simulink model "robust_defence_zda"  (R2022a)
settings: Solver=VariableStepAuto  StartTime=0.0  StopTime=6  RelTol=1e-3
values from neighbouring files (symbols this model uses):
  A = [zeros(3, 3) eye(3) ... (first row only)    [robust_defence_zda.m]
  A_obs1 = [-kappa1*c2   1 0 ... (first row only)    [robust_defence_zda.m]
  A_obs2 = [-kappa2*c2   1 0 ... (first row only)    [robust_defence_zda.m]
  A_obs3 = [-kappa3*c2   1 0 ... (first row only)    [robust_defence_zda.m]
  B = [zeros(3, 3); inv(M)]    [robust_defence_zda.m]
  b = Cp*(A^(r-1))*Bp    [robust_defence_zda.m]
  b0 = 62.5    [robust_defence_zda.m]
  B_obs = [0; b0; 0]    [robust_defence_zda.m]
  Cp = [0 0 1 0 0 0]    [robust_defence_zda.m]
  H0 = Cp*(A^r)*T0_inv    [robust_defence_zda.m]
  K = Cp*(A^r)*T1_inv    [robust_defence_zda.m]
  K0 = [-9 -6]    [robust_defence_zda.m]
  Ka = (-1)*acker(F0, G0a, [1/tau1 1/tau1 1/tau1 1/tau1])    [robust_defence_zda.m]
  kcr1 = [kappa1*c2; kappa1^2*c1; kappa1^3*c0]    [robust_defence_zda.m]
  kcr2 = [kappa2*c2; kappa2^2*c1; kappa2^3*c0]    [robust_defence_zda.m]
  kcr3 = [kappa3*c2; kappa3^2*c1; kappa3^3*c0]    [robust_defence_zda.m]
  L = 0.1    [robust_defence_zda.m]
  T0 = [1 0 0 0 0 0 ... (first row only)    [robust_defence_zda.m]
  T1 = [Cp; Cp*A]    [robust_defence_zda.m]
  x0 = [0; 0; 0; 0; omega20; 0]    [robust_defence_zda.m]
  xi_ext0 = [0; 0.085; 0.01]    [robust_defence_zda.m]
settings Model: Creator=edebi  LastModifiedBy=edebi

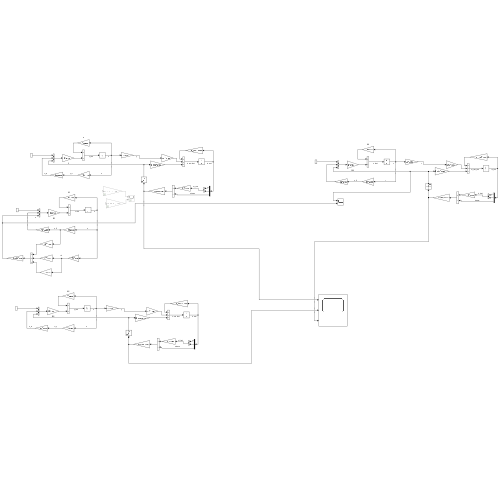
[thumbnail: Simulink's stored preview of the top-level diagram]
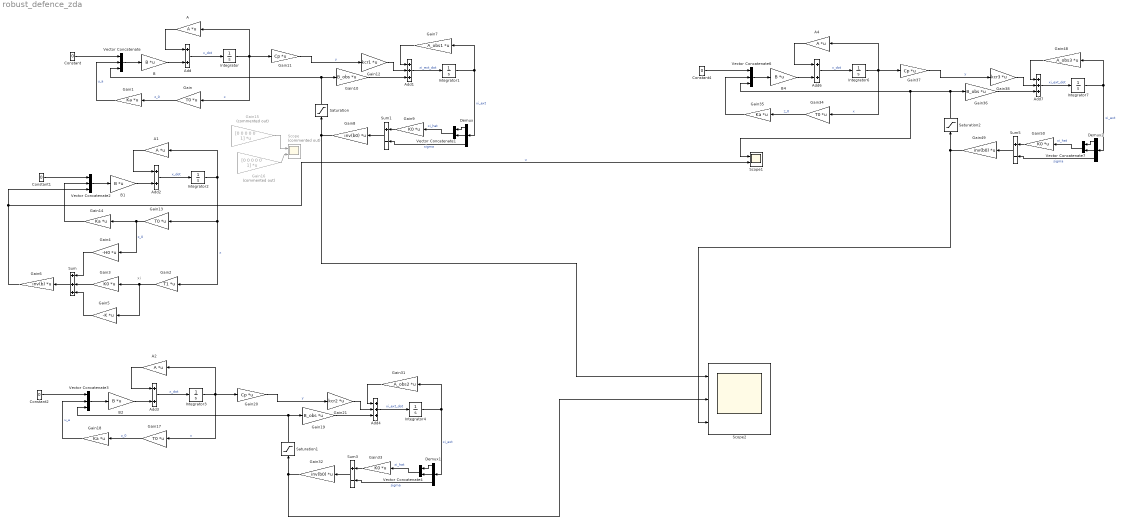
== system robust_defence_zda ==
  note: xi
  A{,1..2,4} (4 alike) : Gain  Gain=A  Multiplication=Matrix(K*u) (u vector)
  Add{,2..3,6} (4 alike) : Sum
  Add1 : Sum  Inputs=+++
  Add4 : Sum  Inputs=+++
  Add7 : Sum  Inputs=+++
  B{,1..2,4} (4 alike) : Gain  Gain=B  Multiplication=Matrix(K*u) (u vector)
  Constant{,1..2,4} (4 alike) : Constant  Value=0
  Demux : Demux  Outputs=3
  Demux1 : Demux  Outputs=3
  Demux2 : Demux  Outputs=3
  Gain{,13,17,34} (4 alike) : Gain  Gain=T0  Multiplication=Matrix(K*u) (u vector)
  Gain{1,14,18,35} (4 alike) : Gain  Gain=Ka  Multiplication=Matrix(K*u) (u vector)
  Gain10 : Gain  Gain=B_obs  Multiplication=Matrix(K*u) (u vector)
  Gain11 : Gain  Gain=Cp  Multiplication=Matrix(K*u) (u vector)
  Gain12 : Gain  Gain=kcr1  Multiplication=Matrix(K*u) (u vector)
  Gain15 : Gain  Commented=on  Gain=[0 0 0 0 0 1]  Multiplication=Matrix(K*u) (u vector)
  Gain16 : Gain  Commented=on  Gain=[0 0 0 0 0 1]  Multiplication=Matrix(K*u) (u vector)
  Gain19 : Gain  Gain=B_obs  Multiplication=Matrix(K*u) (u vector)
  Gain2 : Gain  Gain=T1  Multiplication=Matrix(K*u) (u vector)
  Gain20 : Gain  Gain=Cp  Multiplication=Matrix(K*u) (u vector)
  Gain21 : Gain  Gain=kcr2  Multiplication=Matrix(K*u) (u vector)
  Gain{3,9,33,50} (4 alike) : Gain  Gain=K0  Multiplication=Matrix(K*u) (u vector)
  Gain31 : Gain  Gain=A_obs2  Multiplication=Matrix(K*u) (u vector)
  Gain32 : Gain  Gain=inv(b0)  Multiplication=Matrix(K*u) (u vector)
  Gain36 : Gain  Gain=B_obs  Multiplication=Matrix(K*u) (u vector)
  Gain37 : Gain  Gain=Cp  Multiplication=Matrix(K*u) (u vector)
  Gain38 : Gain  Gain=kcr3  Multiplication=Matrix(K*u) (u vector)
  Gain4 : Gain  Gain=-H0  Multiplication=Matrix(K*u) (u vector)
  Gain48 : Gain  Gain=A_obs3  Multiplication=Matrix(K*u) (u vector)
  Gain49 : Gain  Gain=inv(b0)  Multiplication=Matrix(K*u) (u vector)
  Gain5 : Gain  Gain=-K  Multiplication=Matrix(K*u) (u vector)
  Gain6 : Gain  Gain=inv(b)  Multiplication=Matrix(K*u) (u vector)
  Gain7 : Gain  Gain=A_obs1  Multiplication=Matrix(K*u) (u vector)
  Gain8 : Gain  Gain=inv(b0)  Multiplication=Matrix(K*u) (u vector)
  Integrator{,2..3,6} (4 alike) : Integrator  InitialCondition=x0  ContinuousStateAttributes=['delta1' 'delta2' 'delta3' 'omega1' 'omega2' 'omega3']
  Integrator1 : Integrator  InitialCondition=xi_ext0
  Integrator4 : Integrator  InitialCondition=xi_ext0
  Integrator7 : Integrator  InitialCondition=xi_ext0
  Saturation : Saturate  UpperLimit=+L  LowerLimit=-L
  Saturation1 : Saturate  UpperLimit=+L  LowerLimit=-L
  Saturation2 : Saturate  UpperLimit=+L  LowerLimit=-L
  Scope : Scope  Commented=on  NumInputPorts=2
  Scope1 : Scope  NumInputPorts=2
  Scope2 : Scope  NumInputPorts=3
  Sum : Sum  Inputs=+++
  Sum1 : Sum  Inputs=+-
  Sum3 : Sum  Inputs=+-
  Sum5 : Sum  Inputs=+-
  Vector Concatenate{,2..3,6} (4 alike) : Concatenate  NumInputs=3
  Vector Concatenate1 : Concatenate
  Vector Concatenate4 : Concatenate
  Vector Concatenate7 : Concatenate
  wires:
  Constant/1 -> Vector Concatenate/1
  Sum/1 -> Gain6/1
  Gain5/1 -> Sum/3
  B/1 -> Add/2
  Gain1/1 -> Vector Concatenate/2  "u_a"
  Gain2/1 -> Gain5/1, Gain3/1
  Add/1 -> Integrator/1  "x_dot"
  Gain/1 -> Gain1/1  "z_0"
  Vector Concatenate/1 -> B/1
  Gain3/1 -> Sum/2
  Integrator/1 -> Gain/1, A/1, Gain11/1  "x"
  Gain4/1 -> Sum/1
  A/1 -> Add/1
  Add1/1 -> Integrator1/1  "xi_ext_dot"
  Gain7/1 -> Add1/1
  Demux/3 -> Sum1/2  "sigma"
  Gain9/1 -> Sum1/1
  Sum1/1 -> Gain8/1
  Gain11/1 -> Gain12/1  "y"
  Gain12/1 -> Add1/2
  Integrator1/1 -> Demux/1, Gain7/1  "xi_ext"
  Demux/2 -> Vector Concatenate1/2
  Demux/1 -> Vector Concatenate1/1
  Vector Concatenate1/1 -> Gain9/1  "xi_hat"
  Gain10/1 -> Add1/3
  Gain8/1 -> Saturation/1, Scope2/1
  Saturation/1 -> Gain10/1, Vector Concatenate/3
  Integrator2/1 -> Gain2/1, Gain13/1, A1/1  "x"
  Gain6/1 -> Scope1/2, Vector Concatenate2/3  "u"
  Gain14/1 -> Vector Concatenate2/2
  Gain13/1 -> Gain4/1, Gain14/1  "z_0"
  A1/1 -> Add2/1
  Vector Concatenate2/1 -> B1/1
  Add2/1 -> Integrator2/1  "x_dot"
  B1/1 -> Add2/2
  Constant1/1 -> Vector Concatenate2/1
  Gain15/1 -> Scope/1
  Gain16/1 -> Scope/2
  Gain20/1 -> Gain21/1  "y"
  Integrator4/1 -> Demux1/1, Gain31/1  "xi_ext"
  Add4/1 -> Integrator4/1  "xi_ext_dot"
  Saturation1/1 -> Gain19/1, Vector Concatenate3/3
  Gain19/1 -> Add4/3
  Demux1/2 -> Vector Concatenate4/2
  Demux1/1 -> Vector Concatenate4/1
  Integrator3/1 -> Gain17/1, A2/1, Gain20/1  "x"
  Gain33/1 -> Sum3/1
  Vector Concatenate3/1 -> B2/1
  Gain31/1 -> Add4/1
  Gain17/1 -> Gain18/1  "z_0"
  Gain18/1 -> Vector Concatenate3/2  "u_a"
  A2/1 -> Add3/1
  Gain21/1 -> Add4/2
  Add3/1 -> Integrator3/1  "x_dot"
  Gain32/1 -> Scope2/2, Saturation1/1
  Sum3/1 -> Gain32/1
  Demux1/3 -> Sum3/2  "sigma"
  Vector Concatenate4/1 -> Gain33/1  "xi_hat"
  B2/1 -> Add3/2
  Constant2/1 -> Vector Concatenate3/1
  Gain37/1 -> Gain38/1  "y"
  Integrator7/1 -> Demux2/1, Gain48/1  "xi_ext"
  Add7/1 -> Integrator7/1  "xi_ext_dot"
  Saturation2/1 -> Gain36/1, Scope1/1, Vector Concatenate6/3
  Gain36/1 -> Add7/3
  Demux2/2 -> Vector Concatenate7/2
  Demux2/1 -> Vector Concatenate7/1
  Integrator6/1 -> Gain34/1, A4/1, Gain37/1  "x"
  Gain50/1 -> Sum5/1
  Vector Concatenate6/1 -> B4/1
  Gain48/1 -> Add7/1
  Gain34/1 -> Gain35/1  "z_0"
  Gain35/1 -> Vector Concatenate6/2
  A4/1 -> Add6/1
  Gain38/1 -> Add7/2
  Add6/1 -> Integrator6/1  "x_dot"
  Gain49/1 -> Scope2/3, Saturation2/1
  Sum5/1 -> Gain49/1
  Demux2/3 -> Sum5/2  "sigma"
  Vector Concatenate7/1 -> Gain50/1  "xi_hat"
  B4/1 -> Add6/2
  Constant4/1 -> Vector Concatenate6/1
